simulink model "simulation_three_motors"  (R2023b)
settings: Solver=FixedStepAuto  StartTime=0.0  StopTime=inf  FixedStep=Ts  RelTol=1e-3
libraries: slDxl_lib_old x8
settings Model: Creator=jeihunl  LastModifiedBy=gbiocic
settings SolverCC: AlgebraicLoopSolver=TrustRegion
settings DataIOCC: ReturnWorkspaceOutputs=off
settings OptimizationCC: LifeSpan=inf
settings DebuggingCC: UnconnectedInputMsg=warning  UnconnectedOutputMsg=warning  UnconnectedLineMsg=warning  SFExecutionAtInitializationDiag=none  ArithmeticOperatorsInVariantConditions=warning
settings HardwareCC: ProdBitPerSizeT=32  ProdBitPerPtrDiffT=32  ProdWordSize=32  ProdHWDeviceType=Specified
settings ModelReferenceCC: EnableRefExpFcnMdlSchedulingChecks=on
settings SFSimCC: SimUseLocalCustomCode=off  CustomCodeUndefinedFunction=UseInterfaceOnly
settings RTWCC: RTWUseLocalCustomCode=off
settings CodeAppCC: StateflowObjectComments=on

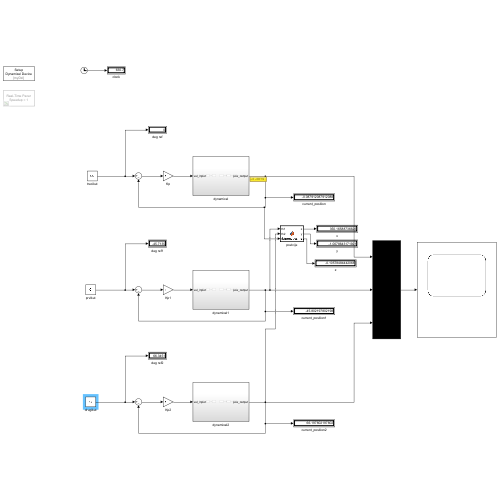
[thumbnail: Simulink's stored preview of the top-level diagram]
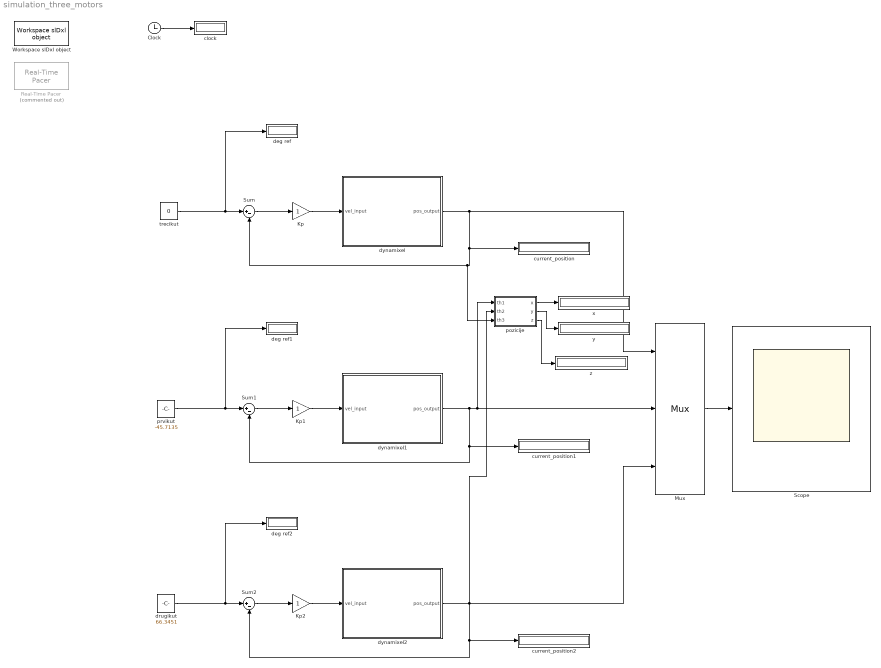
== system simulation_three_motors ==
  Clock : Clock
  Kp : Gain
  Kp1 : Gain
  Kp2 : Gain
  Mux : Mux  Inputs=3
  Real-Time Pacer : slDxl_lib_old/Real-Time Pacer  Commented=on  simTimePerRealTime=1
  Scope : Scope
  Sum : Sum  Inputs=|+-
  Sum1 : Sum  Inputs=|+-
  Sum2 : Sum  Inputs=|+-
  Workspace slDxl object : slDxl_lib_old/Workspace slDxl object  slDxlVarName=Existing Object Handle #1  workspaceVarName=myDxl
  clock : Display
  current_position : Display
      settings: Decimation=5
  current_position1 : Display
      settings: Decimation=5
  current_position2 : Display
      settings: Decimation=5
  deg ref : Display
  deg ref1 : Display
  deg ref2 : Display
  drugikut : Constant  Value=66.3451
  dynamixel : Subsystem
  dynamixel1 : Subsystem
  dynamixel2 : Subsystem
  pozicije : MATLAB Function  TreatAsAtomicUnit=on
  prvikut : Constant  Value=-45.7135
  trecikut : Constant  Value=0
  x : Display
      settings: Decimation=5
  y : Display
      settings: Decimation=5
  z : Display
      settings: Decimation=5
  wires:
  dynamixel/1(pos_output) -> Mux/1, pozicije/3(th3), Sum/2, current_position/1
  Sum/1 -> Kp/1
  trecikut/1 -> deg ref/1, Sum/1
  Clock/1 -> clock/1
  Sum1/1 -> Kp1/1
  prvikut/1 -> deg ref1/1, Sum1/1
  dynamixel1/1(pos_output) -> pozicije/1(th1), Mux/2, Sum1/2, current_position1/1
  Kp1/1 -> dynamixel1/1(vel_input)
  drugikut/1 -> deg ref2/1, Sum2/1
  Kp2/1 -> dynamixel2/1(vel_input)
  dynamixel2/1(pos_output) -> pozicije/2(th2), Mux/3, Sum2/2, current_position2/1
  Sum2/1 -> Kp2/1
  Mux/1 -> Scope/1
  Kp/1 -> dynamixel/1(vel_input)
  pozicije/1(x) -> x/1
  pozicije/2(y) -> y/1
  pozicije/3(z) -> z/1

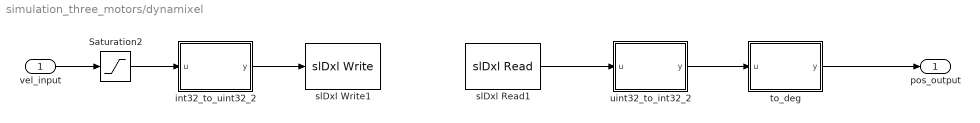
== system simulation_three_motors/dynamixel ==
  vel_input : Inport
  Saturation2 : Saturate  UpperLimit=256  LowerLimit=-256
  int32_to_uint32_2 : MATLAB Function  TreatAsAtomicUnit=on
  slDxl Read1 : slDxl_lib_old/slDxl Read  slDxlObject=Existing Object Handle #1  DXL_ID=1  DXL_ADDR=132  DXL_READ_SIZE=4  sampleT=Ts
  slDxl Write1 : slDxl_lib_old/slDxl Write  slDxlObject=Existing Object Handle #1  DXL_ID=1  DXL_ADDR=104  DXL_WRITE_SIZE=4  sampleT=Ts
  to_deg : MATLAB Function  TreatAsAtomicUnit=on
  uint32_to_int32_2 : MATLAB Function  TreatAsAtomicUnit=on
  pos_output : Outport  VectorParamsAs1DForOutWhenUnconnected=off
  wires:
  vel_input/1 -> Saturation2/1
  uint32_to_int32_2/1(y) -> to_deg/1(u)
  slDxl Read1/1 -> uint32_to_int32_2/1(u)
  Saturation2/1 -> int32_to_uint32_2/1(u)
  to_deg/1(y) -> pos_output/1
  int32_to_uint32_2/1(y) -> slDxl Write1/1

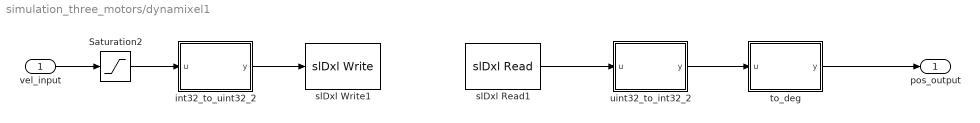
== system simulation_three_motors/dynamixel1 ==
  vel_input : Inport
  Saturation2 : Saturate  UpperLimit=256  LowerLimit=-256
  int32_to_uint32_2 : MATLAB Function  TreatAsAtomicUnit=on
  slDxl Read1 : slDxl_lib_old/slDxl Read  slDxlObject=Existing Object Handle #1  DXL_ID=2  DXL_ADDR=132  DXL_READ_SIZE=4  sampleT=Ts
  slDxl Write1 : slDxl_lib_old/slDxl Write  slDxlObject=Existing Object Handle #1  DXL_ID=2  DXL_ADDR=104  DXL_WRITE_SIZE=4  sampleT=Ts
  to_deg : MATLAB Function  TreatAsAtomicUnit=on
  uint32_to_int32_2 : MATLAB Function  TreatAsAtomicUnit=on
  pos_output : Outport  VectorParamsAs1DForOutWhenUnconnected=off
  wires:
  vel_input/1 -> Saturation2/1
  uint32_to_int32_2/1(y) -> to_deg/1(u)
  slDxl Read1/1 -> uint32_to_int32_2/1(u)
  Saturation2/1 -> int32_to_uint32_2/1(u)
  to_deg/1(y) -> pos_output/1
  int32_to_uint32_2/1(y) -> slDxl Write1/1

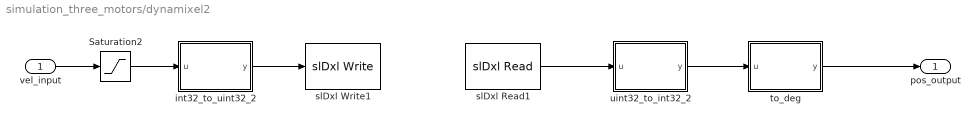
== system simulation_three_motors/dynamixel2 ==
  vel_input : Inport
  Saturation2 : Saturate  UpperLimit=256  LowerLimit=-256
  int32_to_uint32_2 : MATLAB Function  TreatAsAtomicUnit=on
  slDxl Read1 : slDxl_lib_old/slDxl Read  slDxlObject=Existing Object Handle #1  DXL_ID=3  DXL_ADDR=132  DXL_READ_SIZE=4  sampleT=Ts
  slDxl Write1 : slDxl_lib_old/slDxl Write  slDxlObject=Existing Object Handle #1  DXL_ID=3  DXL_ADDR=104  DXL_WRITE_SIZE=4  sampleT=Ts
  to_deg : MATLAB Function  TreatAsAtomicUnit=on
  uint32_to_int32_2 : MATLAB Function  TreatAsAtomicUnit=on
  pos_output : Outport  VectorParamsAs1DForOutWhenUnconnected=off
  wires:
  vel_input/1 -> Saturation2/1
  uint32_to_int32_2/1(y) -> to_deg/1(u)
  slDxl Read1/1 -> uint32_to_int32_2/1(u)
  Saturation2/1 -> int32_to_uint32_2/1(u)
  to_deg/1(y) -> pos_output/1
  int32_to_uint32_2/1(y) -> slDxl Write1/1

== matlab function simulation_three_motors/dynamixel/uint32_to_int32_2 ==
  data: u input; y output
function y = fcn(u)
    temp = typecast(uint32(u), 'int32');
    y = double(temp(1));
end

== matlab function simulation_three_motors/dynamixel1/int32_to_uint32_2 ==
  data: u input; y output
function y = fcn(u)
    temp = typecast(int32(u), 'uint32');
    y = temp(1);
end

== matlab function simulation_three_motors/dynamixel/to_deg ==
  data: u input; y output
function y = fcn(u)
    y = (u / 4095.0) * 360.0;
end

== matlab function simulation_three_motors/dynamixel/int32_to_uint32_2 ==
  data: u input; y output
function y = fcn(u)
    temp = typecast(int32(u), 'uint32');
    y = temp(1);
end

== matlab function simulation_three_motors/dynamixel1/to_deg ==
  data: u input; y output
function y = fcn(u)
    y = (u / 4095.0) * 360.0;
end

== matlab function simulation_three_motors/dynamixel1/uint32_to_int32_2 ==
  data: u input; y output
function y = fcn(u)
    temp = typecast(uint32(u), 'int32');
    y = double(temp(1));
end

== matlab function simulation_three_motors/dynamixel2/int32_to_uint32_2 ==
  data: u input; y output
function y = fcn(u)
    temp = typecast(int32(u), 'uint32');
    y = temp(1);
end

== matlab function simulation_three_motors/dynamixel2/to_deg ==
  data: u input; y output
function y = fcn(u)
    y = (u / 4095.0) * 360.0;
end

== matlab function simulation_three_motors/dynamixel2/uint32_to_int32_2 ==
  data: u input; y output
function y = fcn(u)
    temp = typecast(uint32(u), 'int32');
    y = double(temp(1));
end

== matlab function simulation_three_motors/pozicije ==
  data: x output; th1 input; y output; th2 input; th3 input; z output
function [x, y, z] = direct_kinematics_realtime(th1, th2, th3)
[x, y, z] = direct_kinematics(th1, th2, th3);
end
